simulink model "tracking_1dof_simulink"  (R2020b)
settings: Solver=ode3  StartTime=0.0  StopTime=20  FixedStep=0.01  RelTol=1e-3
settings Model: Creator=Admin  LastModifiedBy=Admin

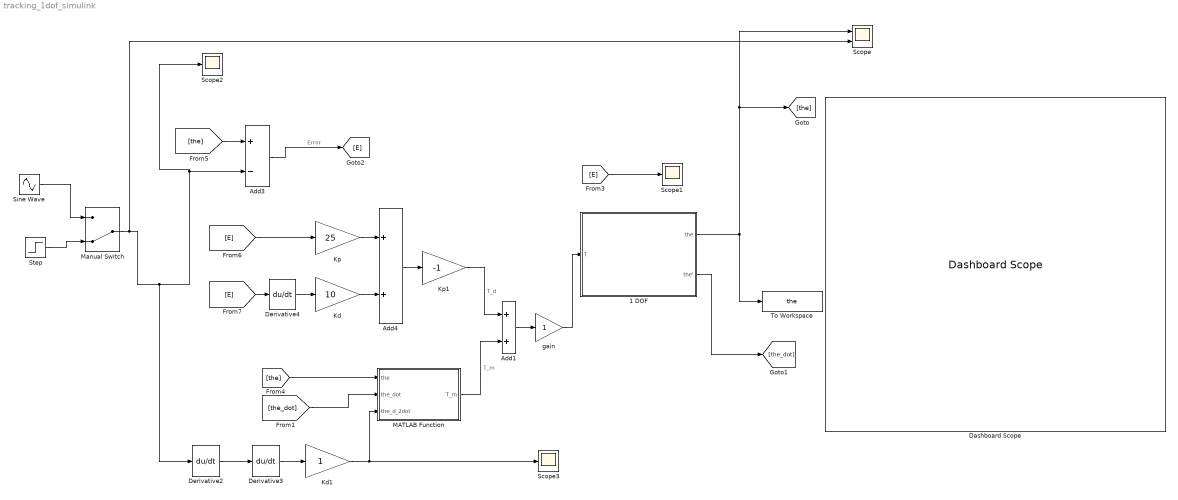
== system tracking_1dof_simulink ==
  1 DOF : Subsystem
  Add1 : Sum
  Add3 : Sum  Inputs=+-
  Add4 : Sum
  Dashboard Scope : DashboardScope
  Derivative2 : Derivative
  Derivative3 : Derivative
  Derivative4 : Derivative
  Kd : Gain  Gain=10
  Kd1 : Gain
  Kp : Gain  Gain=25
  Kp1 : Gain  Gain=-1
  MATLAB Function : MATLAB Function  TreatAsAtomicUnit=on
  Manual Switch : ManualSwitch  CurrentSetting=0
  Scope : Scope  NumInputPorts=2
  Scope1 : Scope
  Scope2 : Scope
  Scope3 : Scope
  Sine Wave : Sin  SampleTime=0
  Step : Step  Time=0  SampleTime=0
  To Workspace : ToWorkspace  VariableName=the  SampleTime=-1
  gain : Gain
  wires:
  1 DOF/2(the') -> [the_dot]
  1 DOF/1(the) -> Scope/1, [the], To Workspace/1
  Add1/1 -> gain/1
  gain/1 -> 1 DOF/1(T)
  Kp1/1 -> Add1/1  "T_d"
  [E] -> Scope1/1
  [the_dot] -> MATLAB Function/2(the_dot)
  [the] -> MATLAB Function/1(the)
  MATLAB Function/1(T_m) -> Add1/2  "T_m"
  [the] -> Add3/1
  Add3/1 -> [E]  "Error"
  [E] -> Kp/1
  [E] -> Derivative4/1
  Derivative4/1 -> Kd/1
  Kd/1 -> Add4/2
  Kp/1 -> Add4/1
  Add4/1 -> Kp1/1
  Derivative2/1 -> Derivative3/1
  Derivative3/1 -> Kd1/1
  Manual Switch/1 -> Scope/2, Scope2/1, Add3/2, Derivative2/1
  Step/1 -> Manual Switch/2
  Kd1/1 -> Scope3/1, MATLAB Function/3(the_d_2dot)
  Sine Wave/1 -> Manual Switch/1

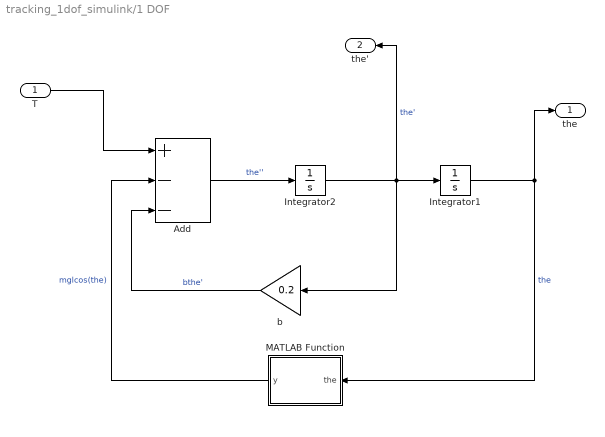
== system tracking_1dof_simulink/1 DOF ==
  T : Inport
  Add : Sum  Inputs=+--
  Integrator1 : Integrator  ZeroCross=off
  Integrator2 : Integrator  ZeroCross=off
  MATLAB Function : MATLAB Function  TreatAsAtomicUnit=on
  b : Gain  Gain=0.2
  the : Outport
  the' : Outport  Port=2
  wires:
  Add/1 -> Integrator2/1  "the''"
  Integrator1/1 -> MATLAB Function/1(the), the/1  "the"
  Integrator2/1 -> the'/1, b/1, Integrator1/1  "the'"
  b/1 -> Add/3  "bthe'"
  MATLAB Function/1(y) -> Add/2  "mglcos(the)"
  T/1 -> Add/1

== matlab function tracking_1dof_simulink/1 DOF/MATLAB Function ==
  data: the input; y output
function y = fcn(the)

y = 9.81*cos(the);

== matlab function tracking_1dof_simulink/MATLAB Function ==
  data: the input; T_m output; the_dot input; the_d_2dot input
function T_m = fcn(the, the_dot, the_d_2dot)


T_m = the_d_2dot + 0.2*the_dot + 9.81*cos(the);
